simulink model "SoftPwmOutputTest"  (R2016a)
settings: Solver=FixedStepAuto  StartTime=0.0  StopTime=10  RelTol=1e-3
settings Model: SimulationMode=external  Creator=Shogo  LastModifiedBy=Shogo
settings SolverCC: PositivePriorityOrder=on
settings DataIOCC: LimitDataPoints=on
settings OptimizationCC: OptimizeModelRefInitCode=on  LifeSpan=1  MaxStackSize=64
settings DebuggingCC: AllowSymbolicDim=off
settings HardwareCC: ProdBitPerPointer=32  ProdLargestAtomicInteger=Long  ProdLargestAtomicFloat=Double  ProdWordSize=32  ProdHWDeviceType=ARM Compatible->ARM Cortex  UseEmbeddedCoderFeatures=off  UseSimulinkCoderFeatures=off
settings ModelReferenceCC: PropagateSignalLabelsOutOfModel=off
settings RTWCC: SystemTargetFile=ert.tlc  HardwareBoard=Raspberry Pi  TemplateMakefile=ert_default_tmf  RTWVerbose=off  Toolchain=GNU GCC Raspberry Pi  IncludeHyperlinkInReport=on
settings CodeAppCC: ForceParamTrailComments=on  OperatorAnnotations=on  SimulinkDataObjDesc=on  SFDataObjDesc=on  MATLABFcnDesc=on  MangleLength=10  InsertBlockDesc=on  MATLABSourceComments=on
settings ERTTargetCC: SupportNonInlinedSFcns=on  SupportVariableSizeSignals=on  ExtMode=on  ExtModeMexArgs='192.168.11.13' 0 17725  ERTSrcFileBannerTemplate=codertarget_code_template.cgt  ERTHdrFileBannerTemplate=codertarget_code_template.cgt  ERTDataSrcFileTemplate=codertarget_code_template.cgt  ERTDataHdrFileTemplate=codertarget_code_template.cgt

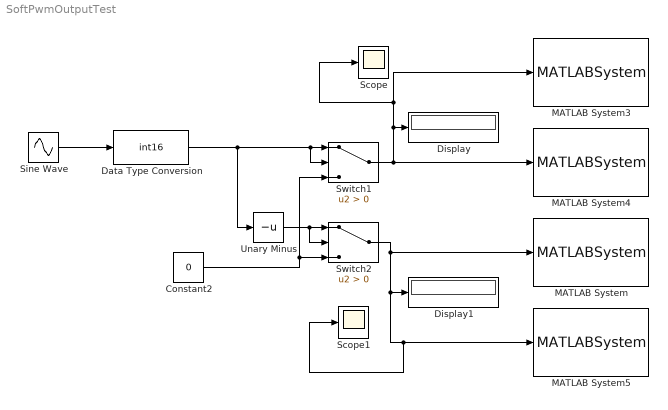
== system SoftPwmOutputTest ==
  Constant2 : Constant  Value=0  OutDataTypeStr=single
  Data Type Conversion : DataTypeConversion  OutDataTypeStr=int16
  Display : Display
  Display1 : Display
  MATLAB System : MATLABSystem  System=SoftPwmOutput  Pin=19  InitialValue=0  PwmRange=100
      mask Type: SoftPwmOutput
      mask Display:
      | disp('SoftPWM Write (19)');
      | port_label('input',1,'u');
  MATLAB System3 : MATLABSystem  System=SoftPwmOutput  Pin=20  InitialValue=0  PwmRange=100
      mask Type: SoftPwmOutput
      mask Display:
      | disp('SoftPWM Write (20)');
      | port_label('input',1,'u');
  MATLAB System4 : MATLABSystem  System=SoftPwmOutput  Pin=21  InitialValue=0  PwmRange=100
      mask Type: SoftPwmOutput
      mask Display:
      | disp('SoftPWM Write (21)');
      | port_label('input',1,'u');
  MATLAB System5 : MATLABSystem  System=SoftPwmOutput  Pin=26  InitialValue=0  PwmRange=100
      mask Type: SoftPwmOutput
      mask Display:
      | disp('SoftPWM Write (26)');
      | port_label('input',1,'u');
  Scope : Scope
  Scope1 : Scope
  Sine Wave : Sin  Amplitude=100  Frequency=5  Phase=pi/2  SampleTime=1
  Switch1 : Switch  Criteria=u2 > Threshold  OutDataTypeStr=uint8
  Switch2 : Switch  Criteria=u2 > Threshold  OutDataTypeStr=uint8
  Unary Minus : UnaryMinus
  wires:
  Sine Wave/1 -> Data Type Conversion/1
  Constant2/1 -> Switch2/3, Switch1/3
  Switch1/1 -> Display/1, MATLAB System3/1, Scope/1, MATLAB System4/1
  Switch2/1 -> Scope1/1, MATLAB System5/1, Display1/1, MATLAB System/1
  Unary Minus/1 -> Switch2/2, Switch2/1
  Data Type Conversion/1 -> Unary Minus/1, Switch1/2, Switch1/1
